simulink model "IdmEstimation_Cogen"  (R2017b)
settings: Solver=FixedStepDiscrete  StartTime=0.0  StopTime=SimTime  FixedStep=0.01  RelTol=1e-3
values from neighbouring files (symbols this model uses):
  BaseMap_CoastAccdiff_Index = (0:0.5:3.5)'    [IdmDev_MdlClassification.m]    (also in IdmParam.mat = [0 0.5 1 1.5 2 2.5 3 3.5])
  BaseMap_CoastSpeed_Index = (5:5:40)'    [IdmDev_MdlClassification.m]    (also in IdmParam.mat = [5 10 15 20 25 30 35 40])
  LrnConfig =     [ModelConfig.mat]
  ModelConfig =     [ModelConfig.mat]
  OnlineConfig =     [ModelConfig.mat]
undefined symbols (not defined in the file or in its folder): acc_veh, dis_veh, ParamCase, vel_veh
libraries: simulink x7
(part 1 of 2)
settings Model: Creator=Kyunghan  LastModifiedBy=Kyunghan
settings DataIOCC: SaveFormat=StructureWithTime
settings OptimizationCC: BlockReduction=off  DefaultParameterBehavior=Inlined  LifeSpan=1
settings DebuggingCC: MultiTaskDSMMsg=warning  FcnCallInpInsideContextMsg=warning  SFExecutionAtInitializationDiag=none
settings HardwareCC: ProdBitPerSizeT=32  ProdBitPerPtrDiffT=32  ProdWordSize=32  ProdHWDeviceType=Specified
settings ModelReferenceCC: PropagateSignalLabelsOutOfModel=off
settings SFSimCC: MATLABDynamicMemAlloc=off
settings RTWCC: SystemTargetFile=ert.tlc  TemplateMakefile=ert_default_tmf  GenerateReport=on  IncludeHyperlinkInReport=on  LaunchReport=on  PortableWordSizes=on  GenerateTraceInfo=on  GenerateTraceReport=on  GenerateTraceReportSl=on  GenerateTraceReportSf=on  GenerateTraceReportEml=on
settings CodeAppCC: ForceParamTrailComments=on  IgnoreCustomStorageClasses=off  OperatorAnnotations=on  SimulinkDataObjDesc=on  SFDataObjDesc=on  InsertBlockDesc=on  StateflowObjectComments=on
settings ERTTargetCC: MultiwordLength=2048  GenerateSampleERTMain=on  MultiInstanceERTCode=on  CodeInterfacePackaging=Reusable function  SupportContinuousTime=on  SupportVariableSizeSignals=on  InlinedParameterPlacement=NonHierarchical  MultiInstanceErrorCode=Warning  RootIOFormat=Structure reference  ERTCustomFileTemplate=example_file_process.tlc  EnableDataOwnership=on  GlobalDataDefinition=InSeparateSourceFile  DataDefinitionFile=Idm_Param.c  GlobalDataReference=InSeparateHeaderFile  DataReferenceFile=Idm_Param.h  ConvertIfToSwitch=off  SuppressUnreachableDefaultCases=off

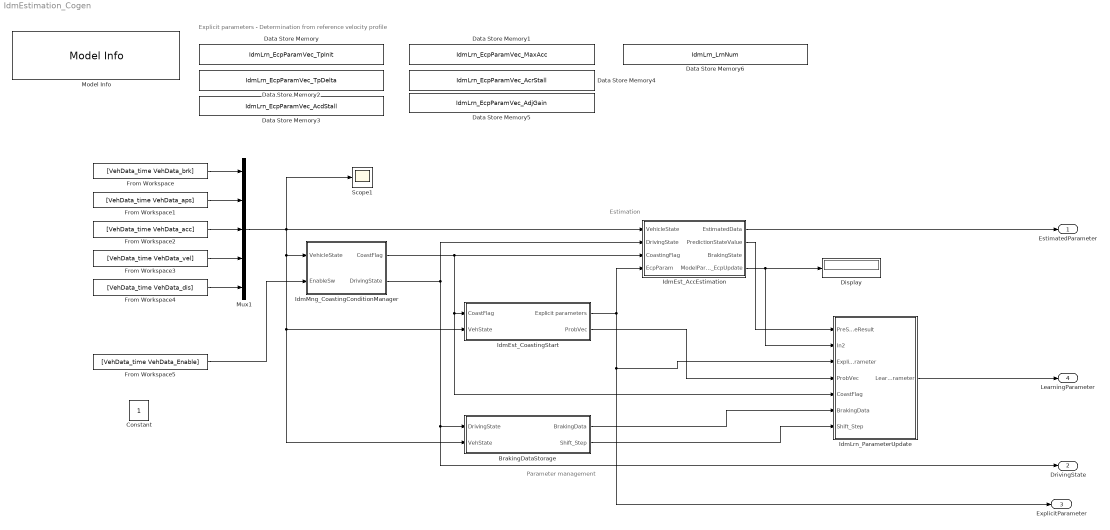
== system IdmEstimation_Cogen ==
  note: Parameter management
  note: Estimation
  note: Explicit parameters - Determination from reference velocity profile
  BrakingDataStorage : Subsystem
      settings: RTWFcnNameOpts=Use subsystem name  RTWFileNameOpts=Use subsystem name
  Constant : Constant  OutDataTypeStr=single
  Data Store Memory : DataStoreMemory  DataStoreName=IdmLrn_EcpParamVec_TpInit  ReadBeforeWriteMsg=warning  WriteAfterWriteMsg=warning  WriteAfterReadMsg=warning  InitialValue=BaseMap_TpShift_Data  ShowAdditionalParam=off  Dimensions=LrnConfig.DataIndexLength  StateMustResolveToSignalObject=on
  Data Store Memory1 : DataStoreMemory  DataStoreName=IdmLrn_EcpParamVec_MaxAcc  ReadBeforeWriteMsg=warning  WriteAfterWriteMsg=warning  WriteAfterReadMsg=warning  InitialValue=BaseMap_MaxAcc_Data  ShowAdditionalParam=off  Dimensions=LrnConfig.DataIndexLength  StateMustResolveToSignalObject=on
  Data Store Memory2 : DataStoreMemory  DataStoreName=IdmLrn_EcpParamVec_TpDelta  ReadBeforeWriteMsg=warning  WriteAfterWriteMsg=warning  WriteAfterReadMsg=warning  InitialValue=BaseMap_TpDelta_Data  ShowAdditionalParam=off  Dimensions=LrnConfig.DataIndexLength  StateMustResolveToSignalObject=on
  Data Store Memory3 : DataStoreMemory  DataStoreName=IdmLrn_EcpParamVec_AcdStall  ReadBeforeWriteMsg=warning  WriteAfterWriteMsg=warning  WriteAfterReadMsg=warning  InitialValue=BaseMap_AccDiff_Data  ShowAdditionalParam=off  Dimensions=LrnConfig.DataIndexLength  StateMustResolveToSignalObject=on
  Data Store Memory4 : DataStoreMemory  DataStoreName=IdmLrn_EcpParamVec_AcrStall  ReadBeforeWriteMsg=warning  WriteAfterWriteMsg=warning  WriteAfterReadMsg=warning  InitialValue=BaseMap_AprStall_Data  ShowAdditionalParam=off  Dimensions=LrnConfig.DataIndexLength  StateMustResolveToSignalObject=on
  Data Store Memory5 : DataStoreMemory  DataStoreName=IdmLrn_EcpParamVec_AdjGain  ReadBeforeWriteMsg=warning  WriteAfterWriteMsg=warning  WriteAfterReadMsg=warning  InitialValue=BaseMap_AdjGain_Data  ShowAdditionalParam=off  Dimensions=LrnConfig.DataIndexLength  StateMustResolveToSignalObject=on
  Data Store Memory6 : DataStoreMemory  DataStoreName=IdmLrn_LrnNum  ReadBeforeWriteMsg=warning  WriteAfterWriteMsg=warning  WriteAfterReadMsg=warning  InitialValue=LrnFacNum  ShowAdditionalParam=off  Dimensions=1  StateMustResolveToSignalObject=on
  Display : Display
  From Workspace : FromWorkspace  VariableName=[VehData_time VehData_brk]  SampleTime=0.01
  From Workspace1 : FromWorkspace  VariableName=[VehData_time VehData_aps]  SampleTime=0.01
  From Workspace2 : FromWorkspace  VariableName=[VehData_time VehData_acc]  SampleTime=0.01
  From Workspace3 : FromWorkspace  VariableName=[VehData_time VehData_vel]  SampleTime=0.01
  From Workspace4 : FromWorkspace  VariableName=[VehData_time VehData_dis]  SampleTime=0.01
  From Workspace5 : FromWorkspace  VariableName=[VehData_time VehData_Enable]  SampleTime=0.01
  IdmEst_AccEstimation : Subsystem
      settings: RTWFcnNameOpts=Use subsystem name  RTWFileNameOpts=Use subsystem name
  IdmEst_CoastingStart : Subsystem
      settings: RTWFcnNameOpts=Use subsystem name  RTWFileNameOpts=Use subsystem name
  IdmLrn_ParameterUpdate : Subsystem
      settings: RTWFcnNameOpts=Use subsystem name  RTWFileNameOpts=Use subsystem name
  IdmMng_CoastingConditionManager : Subsystem
      settings: RTWFcnNameOpts=Use subsystem name  RTWFileNameOpts=Use subsystem name
  Model Info : simulink/Model-Wide Utilities/Model Info  Frame=on  DisplayStringWithTags=|  HorizontalTextAlignment=Left  LeftAlignmentValue=0.02
      | * Model description: %<Description>
      |   1. Description: Estimation model of Idm ver 2
      |   2. Created %<Created> by Kyunghan
      |   3. Modfied %<ModifiedDate> by Kyunghan 
      |   4. Model version:  Ver. 2
  Mux1 : Mux  Inputs=5
  Scope1 : Scope
  EstimatedParameter : Outport
  DrivingState : Outport  Port=2
  ExplicitParameter : Outport  Port=3
  LearningParameter : Outport  Port=4
  wires:
  IdmEst_CoastingStart/1(Explicit parameters) -> IdmEst_AccEstimation/4(EcpParam), ExplicitParameter/1, IdmLrn_ParameterUpdate/3(Explicit parameter)
  Mux1/1 -> Scope1/1, IdmEst_AccEstimation/1(VehicleState), IdmEst_CoastingStart/2(VehState), BrakingDataStorage/2(VehState), IdmMng_CoastingConditionManager/1(VehicleState)
  IdmMng_CoastingConditionManager/1(CoastFlag) -> IdmEst_AccEstimation/3(CoastingFlag), IdmEst_CoastingStart/1(CoastFlag), IdmLrn_ParameterUpdate/5(CoastFlag)
  IdmMng_CoastingConditionManager/2(DrivingState) -> IdmEst_AccEstimation/2(DrivingState), DrivingState/1, BrakingDataStorage/1(DrivingState)
  IdmEst_AccEstimation/1(EstimatedData) -> EstimatedParameter/1
  IdmEst_CoastingStart/2(ProbVec) -> IdmLrn_ParameterUpdate/4(ProbVec)
  BrakingDataStorage/1(BrakingData) -> IdmLrn_ParameterUpdate/6(BrakingData)
  IdmLrn_ParameterUpdate/1(LearningParameter) -> LearningParameter/1
  From Workspace1/1 -> Mux1/2
  From Workspace2/1 -> Mux1/3
  From Workspace/1 -> Mux1/1
  From Workspace3/1 -> Mux1/4
  From Workspace4/1 -> Mux1/5
  IdmEst_AccEstimation/2(PredictionStateValue) -> IdmLrn_ParameterUpdate/1(PreStateResult)
  From Workspace5/1 -> IdmMng_CoastingConditionManager/2(EnableSw)
  IdmEst_AccEstimation/4(ModelParam_EcpUpdate) -> Display/1, IdmLrn_ParameterUpdate/2(In2)
  BrakingDataStorage/2(Shift_Step) -> IdmLrn_ParameterUpdate/7(Shift_Step)

== system IdmEstimation_Cogen/BrakingDataStorage ==
  DrivingState : Inport
  VehState : Inport  Port=2
  Compare To Constant1 : simulink/Logic and Bit Operations/Compare To Constant  relop===  const=OnlineConfig.DriveState.Braking  OutDataTypeStr=boolean
  Start state : Subsystem
  BrakingData : Outport
  Shift_Step : Outport  Port=2
  wires:
  Start state/1(BrakingData) -> BrakingData/1
  DrivingState/1 -> Compare To Constant1/1
  VehState/1 -> Start state/1(veh_state)
  Compare To Constant1/1 -> Start state/Enable
  Start state/2(Out1) -> Shift_Step/1

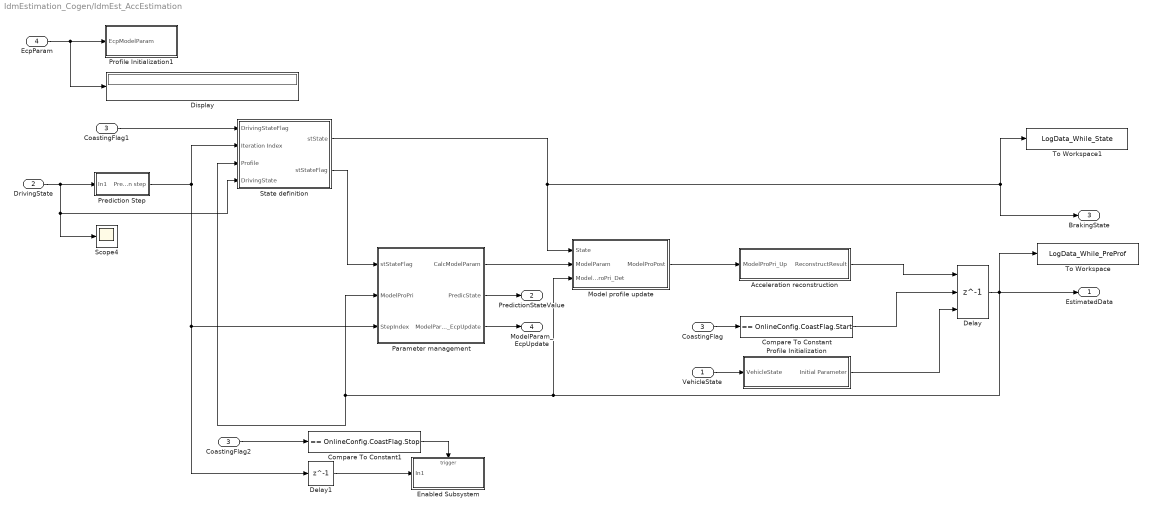
== system IdmEstimation_Cogen/IdmEst_AccEstimation ==
  VehicleState : Inport
  DrivingState : Inport  Port=2
  CoastingFlag : Inport  Port=3
  EcpParam : Inport  Port=4
  Acceleration reconstruction : Subsystem
  CoastingFlag1 : InportShadow  Port=3
  CoastingFlag2 : InportShadow  Port=3
  Compare To Constant : simulink/Logic and Bit Operations/Compare To Constant  relop===  const=OnlineConfig.CoastFlag.Start  OutDataTypeStr=boolean
  Compare To Constant1 : simulink/Logic and Bit Operations/Compare To Constant  relop===  const=OnlineConfig.CoastFlag.Stop  OutDataTypeStr=boolean
  Delay : Delay  DelayLength=1  InitialConditionSource=Input port  InitialCondition=[acc_veh(1) 0 vel_veh(1) vel_veh(1)-ParamCase.VpDiff_Coast dis_veh(1) 0 0]  ExternalReset=Rising
      settings: InputPortMap=u0,r5,p4
  Delay1 : Delay  DelayLength=1
  Display : Display
  Enabled Subsystem : Subsystem  TreatAsAtomicUnit=on
  Model profile update : Subsystem
  Parameter management : Subsystem
  Prediction Step : Subsystem
  Profile Initialization : Subsystem
  Profile Initialization1 : Subsystem
  Scope4 : Scope
  State definition : Subsystem
  To Workspace : ToWorkspace  VariableName=LogData_While_PreProf  SaveFormat=Structure With Time  SampleTime=-1
  To Workspace1 : ToWorkspace  VariableName=LogData_While_State  SaveFormat=Structure With Time  SampleTime=-1
  EstimatedData : Outport  InitialOutput=zeros(1,7)
  PredictionStateValue : Outport  Port=2  InitialOutput=zeros(1,6)
  BrakingState : Outport  Port=3
  ModelParam_EcpUpdate : Outport  Port=4
  wires:
  Compare To Constant/1 -> Delay/2
  Prediction Step/1(Prediction step) -> State definition/2(Iteration Index), Delay1/1, Parameter management/3(StepIndex)
  State definition/2(stStateFlag) -> Parameter management/1(stStateFlag)
  Delay/1 -> To Workspace/1, EstimatedData/1, Model profile update/3(ModelProPri_Det), Parameter management/2(ModelProPri), State definition/3(Profile)
  EcpParam/1 -> Display/1, Profile Initialization1/1(EcpModelParam)
  VehicleState/1 -> Profile Initialization/1(VehicleState)
  Parameter management/1(CalcModelParam) -> Model profile update/2(ModelParam)
  Acceleration reconstruction/1(ReconstructResult) -> Delay/1
  Model profile update/1(ModelProPost) -> Acceleration reconstruction/1(ModelProPri_Up)
  Profile Initialization/1(Initial Parameter) -> Delay/3
  State definition/1(stState) -> BrakingState/1, To Workspace1/1, Model profile update/1(State)
  DrivingState/1 -> State definition/4(DrivingState), Scope4/1, Prediction Step/1(In1)
  Parameter management/2(PredicState) -> PredictionStateValue/1
  CoastingFlag/1 -> Compare To Constant/1
  CoastingFlag1/1 -> State definition/1(DrivingStateFlag)
  Parameter management/3(ModelParam_EcpUpdate) -> ModelParam_EcpUpdate/1
  CoastingFlag2/1 -> Compare To Constant1/1
  Compare To Constant1/1 -> Enabled Subsystem/Trigger
  Delay1/1 -> Enabled Subsystem/1(In1)

== system IdmEstimation_Cogen/IdmEst_CoastingStart ==
  CoastFlag : Inport
  VehState : Inport  Port=2
  Compare To Constant : simulink/Logic and Bit Operations/Compare To Constant  relop===  const=OnlineConfig.CoastFlag.Start  OutDataTypeStr=boolean
  Explicit parameter selection : Subsystem
  Explicit parameters : Outport
  ProbVec : Outport  Port=2
  wires:
  Explicit parameter selection/1(ExplicitParameter) -> Explicit parameters/1
  CoastFlag/1 -> Compare To Constant/1
  VehState/1 -> Explicit parameter selection/1(VehicleState)
  Compare To Constant/1 -> Explicit parameter selection/Trigger
  Explicit parameter selection/2(ProbVec_vel) -> ProbVec/1

== system IdmEstimation_Cogen/IdmLrn_ParameterUpdate ==
  PreStateResult : Inport
  In2 : Inport  Port=2
  Explicit parameter : Inport  Port=3
  ProbVec : Inport  Port=4
  CoastFlag : Inport  Port=5
  BrakingData : Inport  Port=6
  Shift_Step : Inport  Port=7
  Compare To Constant : simulink/Logic and Bit Operations/Compare To Constant  relop===  const=OnlineConfig.CoastFlag.Stop  OutDataTypeStr=boolean
  Compare To Constant1 : simulink/Logic and Bit Operations/Compare To Constant  relop===  const=OnlineConfig.CoastFlag.Stop  OutDataTypeStr=boolean
  End state : Subsystem
  Parameter update : Subsystem
  LearningParameter : Outport
  wires:
  Compare To Constant/1 -> Parameter update/Trigger
  Explicit parameter/1 -> Parameter update/1(ExplicitParameter)
  ProbVec/1 -> Parameter update/3(ProbVec)
  End state/1(LearningParameter) -> Parameter update/2(LearningParameter), LearningParameter/1
  CoastFlag/1 -> Compare To Constant1/1, Compare To Constant/1
  Compare To Constant1/1 -> End state/Trigger
  BrakingData/1 -> End state/1(BrakingDataArry)
  PreStateResult/1 -> Parameter update/4(PreStateResult), End state/3(PreStateResult)
  In2/1 -> Parameter update/5(In5)
  Shift_Step/1 -> End state/2(Shift_Step)

== system IdmEstimation_Cogen/IdmMng_CoastingConditionManager ==
  VehicleState : Inport
  EnableSw : Inport  Port=2
  Chart : Stateflow chart  TreatAsAtomicUnit=on
  Constant : Constant  Value=0
  Selector : Selector  InputPortWidth=OnlineConfig.VehStateSize  IndexOptions=Index vector (dialog)  Indices=OnlineConfig.VehStateIndex.Aps  OutputSizes=1
  Selector1 : Selector  InputPortWidth=OnlineConfig.VehStateSize  IndexOptions=Index vector (dialog)  Indices=OnlineConfig.VehStateIndex.Vel  OutputSizes=1
  Selector2 : Selector  InputPortWidth=OnlineConfig.VehStateSize  IndexOptions=Index vector (dialog)  Indices=OnlineConfig.VehStateIndex.Dis  OutputSizes=1
  Switch : Switch  Threshold=0.5
  Switch1 : Switch  Threshold=0.5
  CoastFlag : Outport
  DrivingState : Outport  Port=2
  wires:
  VehicleState/1 -> Selector2/1, Selector1/1, Selector/1
  Selector/1 -> Chart/1(Aps)
  Selector1/1 -> Chart/2(Vel)
  Chart/2(stCoastFlag) -> Switch1/1
  Chart/1(stDrvState) -> Switch/1
  Selector2/1 -> Chart/3(Dis)
  EnableSw/1 -> Switch1/2, Switch/2
  Switch/1 -> DrivingState/1
  Constant/1 -> Switch/3, Switch1/3
  Switch1/1 -> CoastFlag/1

== system IdmEstimation_Cogen/BrakingDataStorage/Start state ==
  veh_state : Inport
  Enable : EnablePort  StatesWhenEnabling=reset
  MATLAB Function : MATLAB Function  TreatAsAtomicUnit=on
  MATLAB Function1 : MATLAB Function  TreatAsAtomicUnit=on
  Scope : Scope
  Scope1 : Scope
  Selector : Selector  InputPortWidth=5  IndexOptions=Index vector (dialog)  Indices=1  OutputSizes=1
  BrakingData : Outport  InitialOutput=zeros(2000,3)
  Out1 : Outport  Port=2
  wires:
  MATLAB Function/1(BrakingDataOut) -> BrakingData/1
  veh_state/1 -> Selector/1, MATLAB Function/1(veh_state)
  Selector/1 -> Scope/1, MATLAB Function1/1(Brk_Data)
  MATLAB Function1/1(Shift_TimeOut) -> Scope1/1, Out1/1

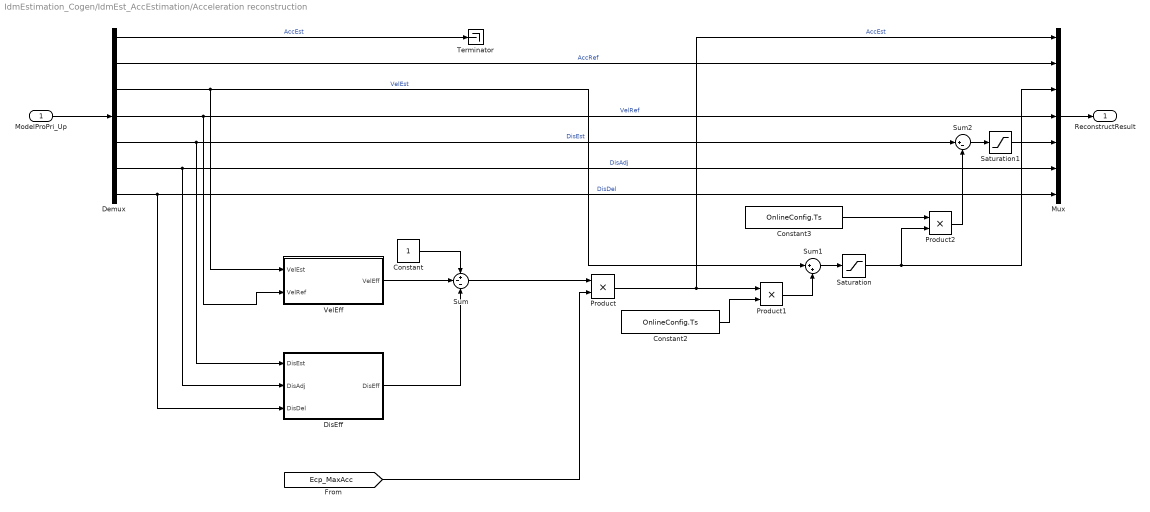
== system IdmEstimation_Cogen/IdmEst_AccEstimation/Acceleration reconstruction ==
  ModelProPri_Up : Inport
  Constant : Constant
  Constant2 : Constant  Value=OnlineConfig.Ts
  Constant3 : Constant  Value=OnlineConfig.Ts
  Demux : Demux  Outputs=7
  DisEff : Subsystem
  Mux : Mux  Inputs=7
  Product : Product
  Product1 : Product
  Product2 : Product
  Saturation : Saturate  UpperLimit=inf  LowerLimit=0.01
  Saturation1 : Saturate  UpperLimit=inf  LowerLimit=0.5001
  Sum : Sum  Inputs=+--
  Sum1 : Sum  Inputs=|++
  Sum2 : Sum  Inputs=|+-
  Terminator : Terminator
  VelEff : Subsystem
  ReconstructResult : Outport
  wires:
  ModelProPri_Up/1 -> Demux/1
  Demux/2 -> Mux/2  "AccRef"
  Mux/1 -> ReconstructResult/1
  Demux/5 -> DisEff/1(DisEst), Sum2/1  "DisEst"
  Demux/6 -> DisEff/2(DisAdj), Mux/6  "DisAdj"
  Demux/7 -> DisEff/3(DisDel), Mux/7  "DisDel"
  Demux/3 -> VelEff/1(VelEst), Sum1/1  "VelEst"
  Demux/4 -> VelEff/2(VelRef), Mux/4  "VelRef"
  VelEff/1(VelEff) -> Sum/2
  DisEff/1(DisEff) -> Sum/3
  Constant/1 -> Sum/1
  Sum/1 -> Product/1
  [Ecp_MaxAcc] -> Product/2
  Product/1 -> Mux/1, Product1/1  "AccEst"
  Constant2/1 -> Product1/2
  Product1/1 -> Sum1/2
  Sum1/1 -> Saturation/1
  Demux/1 -> Terminator/1  "AccEst"
  Constant3/1 -> Product2/1
  Product2/1 -> Sum2/2
  Sum2/1 -> Saturation1/1
  Saturation/1 -> Product2/2, Mux/3
  Saturation1/1 -> Mux/5

== system IdmEstimation_Cogen/IdmEst_AccEstimation/Enabled Subsystem ==
  In1 : Inport
  Trigger : TriggerPort  VariantControl=Variant  PortDimensions=1
  To Workspace : ToWorkspace  VariableName=LogData_Stop_PreSize  SaveFormat=Structure With Time  SampleTime=-1
  wires:
  In1/1 -> To Workspace/1

== system IdmEstimation_Cogen/IdmEst_AccEstimation/Model profile update ==
  State : Inport
  ModelParam : Inport  Port=2
  ModelProPri_Det : Inport  Port=3
  If : If  IfExpression=u1 == 1  ElseIfExpressions=u1 == 2, u1 == 3, u1 == 4, u1 == 5
  Merge : Merge  Inputs=6
  Model profile update - Coast state : Subsystem
  Model profile update - Disadj state : Subsystem
  Model profile update - Initial state : Subsystem
  Model profile update - Term state : Subsystem
  Model profile update - Term state1 : Subsystem
  Model profile update - Veladj state : Subsystem
  ModelProPost : Outport
  wires:
  ModelProPri_Det/1 -> Model profile update - Coast state/1(ModProfPri), Model profile update - Term state1/1(ModProfPri), Model profile update - Term state/1(ModProfPri), Model profile update - Disadj state/1(ModProfPri), Model profile update - Veladj state/1(ModProfPri), Model profile update - Initial state/1(ModProfPri)
  ModelParam/1 -> Model profile update - Initial state/2(ModParam), Model profile update - Veladj state/2(ModParam), Model profile update - Term state/2(ModParam), Model profile update - Disadj state/2(ModParam)
  Merge/1 -> ModelProPost/1
  State/1 -> If/1
  If/4 -> Model profile update - Disadj state/Action
  If/1 -> Model profile update - Coast state/Action
  If/5 -> Model profile update - Term state/Action
  If/2 -> Model profile update - Initial state/Action
  If/3 -> Model profile update - Veladj state/Action
  Model profile update - Coast state/1(ModProf) -> Merge/1
  Model profile update - Initial state/1(ModProf) -> Merge/2
  Model profile update - Veladj state/1(ModProf) -> Merge/3
  Model profile update - Disadj state/1(ModProf) -> Merge/4
  Model profile update - Term state/1(ModProf) -> Merge/5
  If/6 -> Model profile update - Term state1/Action
  Model profile update - Term state1/1(ModProf) -> Merge/6
  [Ecp_AdjGain] -> Model profile update - Disadj state/3(EcpParam_AdjGain)

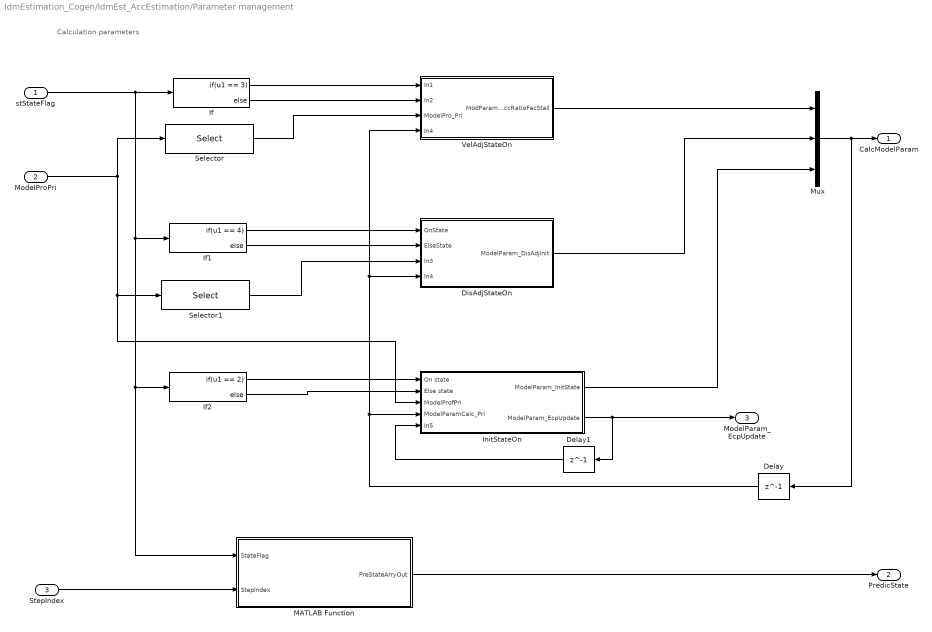
== system IdmEstimation_Cogen/IdmEst_AccEstimation/Parameter management ==
  note: Calculation parameters
  stStateFlag : Inport
  ModelProPri : Inport  Port=2
  StepIndex : Inport  Port=3
  Delay : Delay  DelayLength=1
  Delay1 : Delay  DelayLength=1
  DisAdjStateOn : Subsystem
  If : If  IfExpression=u1 == 3
  If1 : If  IfExpression=u1 == 4
  If2 : If  IfExpression=u1 == 2
  InitStateOn : Subsystem
  MATLAB Function : MATLAB Function  TreatAsAtomicUnit=on
  Mux : Mux  Inputs=3
  Selector : Selector  InputPortWidth=7  IndexOptions=Index vector (dialog)  Indices=[1 3 5]  OutputSizes=1
  Selector1 : Selector  InputPortWidth=7  IndexOptions=Index vector (dialog)  Indices=[1 2]  OutputSizes=1
  VelAdjStateOn : Subsystem
  CalcModelParam : Outport
  PredicState : Outport  Port=2
  ModelParam_EcpUpdate : Outport  Port=3
  wires:
  stStateFlag/1 -> If2/1, MATLAB Function/1(StateFlag), If1/1, If/1
  Mux/1 -> Delay/1, CalcModelParam/1
  Delay/1 -> InitStateOn/4(ModelParamCalc_Pri), VelAdjStateOn/4(In4), DisAdjStateOn/4(In4)
  If2/1 -> InitStateOn/1(On state)
  If2/2 -> InitStateOn/2(Else state)
  ModelProPri/1 -> InitStateOn/3(ModelProfPri), Selector1/1, Selector/1
  InitStateOn/1(ModelParam_InitState) -> Mux/3
  If1/1 -> DisAdjStateOn/1(OnState)
  If1/2 -> DisAdjStateOn/2(ElseState)
  Selector1/1 -> DisAdjStateOn/3(In3)
  DisAdjStateOn/1(ModelParam_DisAdjInit) -> Mux/2
  If/1 -> VelAdjStateOn/1(In1)
  If/2 -> VelAdjStateOn/2(In2)
  Selector/1 -> VelAdjStateOn/3(ModelPro_Pri)
  VelAdjStateOn/1(ModParam_AccRatioFacStall) -> Mux/1
  StepIndex/1 -> MATLAB Function/2(StepIndex)
  MATLAB Function/1(PreStateArryOut) -> PredicState/1
  InitStateOn/2(ModelParam_EcpUpdate) -> ModelParam_EcpUpdate/1, Delay1/1
  Delay1/1 -> InitStateOn/5(In5)

== system IdmEstimation_Cogen/IdmEst_AccEstimation/Prediction Step ==
  In1 : Inport
  Delay : Delay  DelayLength=1
  If : If  IfExpression=u1 == 1
  If Action Subsystem : Subsystem  TreatAsAtomicUnit=on
  If Action Subsystem1 : Subsystem  TreatAsAtomicUnit=on
  Merge : Merge
  Prediction step : Outport
  wires:
  If/1 -> If Action Subsystem/Action
  If/2 -> If Action Subsystem1/Action
  If Action Subsystem/1(Out1) -> Merge/1
  If Action Subsystem1/1(Out1) -> Merge/2
  Merge/1 -> Prediction step/1, Delay/1
  In1/1 -> If/1
  Delay/1 -> If Action Subsystem/1(In1)

== system IdmEstimation_Cogen/IdmEst_AccEstimation/Profile Initialization ==
  VehicleState : Inport
  Constant : Constant  Value=0
  Constant2 : Constant  Value=0
  Constant3 : Constant  Value=0
  Mux : Mux  Inputs=7
  Selector1 : Selector  InputPortWidth=OnlineConfig.VehStateSize  IndexOptions=Index vector (dialog)  Indices=OnlineConfig.VehStateIndex.Vel  OutputSizes=1
  Selector2 : Selector  InputPortWidth=OnlineConfig.VehStateSize  IndexOptions=Index vector (dialog)  Indices=OnlineConfig.VehStateIndex.Dis  OutputSizes=1
  Selector3 : Selector  InputPortWidth=OnlineConfig.VehStateSize  IndexOptions=Index vector (dialog)  Indices=OnlineConfig.VehStateIndex.Acc  OutputSizes=1
  Subsystem : Subsystem
  Initial Parameter : Outport
  wires:
  Constant/1 -> Mux/2
  Subsystem/1(VelRefInit) -> Mux/4
  Constant2/1 -> Mux/6
  Constant3/1 -> Mux/7
  VehicleState/1 -> Selector3/1, Selector2/1, Selector1/1
  Mux/1 -> Initial Parameter/1
  Selector2/1 -> Mux/5
  Selector1/1 -> Subsystem/1(Vel), Mux/3
  Selector3/1 -> Subsystem/2(Acc), Mux/1

== system IdmEstimation_Cogen/IdmEst_AccEstimation/Profile Initialization1 ==
  EcpModelParam : Inport
  Selector : Selector  InputPortWidth=OnlineConfig.EpcParamSize  IndexOptions=Index vector (dialog)  Indices=OnlineConfig.EpcParamIndex.TpInit  OutputSizes=1
  Selector1 : Selector  InputPortWidth=OnlineConfig.EpcParamSize  IndexOptions=Index vector (dialog)  Indices=OnlineConfig.EpcParamIndex.TpStall  OutputSizes=1
  Selector3 : Selector  InputPortWidth=OnlineConfig.EpcParamSize  IndexOptions=Index vector (dialog)  Indices=OnlineConfig.EpcParamIndex.AcrStall  OutputSizes=1
  Selector4 : Selector  InputPortWidth=OnlineConfig.EpcParamSize  IndexOptions=Index vector (dialog)  Indices=OnlineConfig.EpcParamIndex.AccMax  OutputSizes=1
  Selector5 : Selector  InputPortWidth=OnlineConfig.EpcParamSize  IndexOptions=Index vector (dialog)  Indices=OnlineConfig.EpcParamIndex.AdjGain  OutputSizes=1
  tag scope: Ecp_AdjGain=global, Ecp_ArStall=global, Ecp_MaxAcc=global, Ecp_TpDelta=global, Ecp_TpInit=global
  wires:
  EcpModelParam/1 -> Selector1/1, Selector5/1, Selector4/1, Selector3/1, Selector/1
  Selector/1 -> [Ecp_TpInit]
  Selector3/1 -> [Ecp_ArStall]
  Selector1/1 -> [Ecp_TpDelta]
  Selector4/1 -> [Ecp_MaxAcc]
  Selector5/1 -> [Ecp_AdjGain]

== system IdmEstimation_Cogen/IdmEst_AccEstimation/State definition ==
  DrivingStateFlag : Inport
  Iteration Index : Inport  Port=2
  Profile : Inport  Port=3
  DrivingState : Inport  Port=4
  Chart : Stateflow chart  TreatAsAtomicUnit=on
  stState : Outport
  stStateFlag : Outport  Port=2
  wires:
  Profile/1 -> Chart/4(ModelProfile)
  Iteration Index/1 -> Chart/3(IndexTimeStep)
  Chart/1(stState) -> stState/1
  Chart/2(stStateFlag) -> stStateFlag/1
  [Ecp_TpInit] -> Chart/5(Param_Tp_Init)
  [Ecp_TpDelta] -> Chart/6(Param_Tp_Delta)
  [Ecp_ArStall] -> Chart/7(Param_Acr_Stall)
  DrivingStateFlag/1 -> Chart/1(DrvStateFlag)
  DrivingState/1 -> Chart/2(DrivingState)

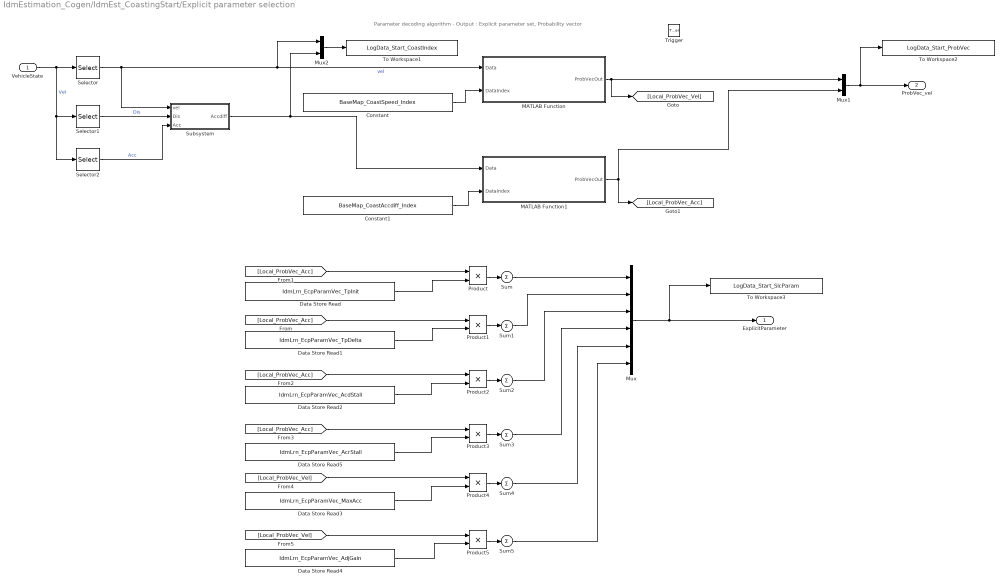
== system IdmEstimation_Cogen/IdmEst_CoastingStart/Explicit parameter selection ==
  note: Parameter decoding algorithm - Output : Explicit parameter set, Probability vector
  VehicleState : Inport
  Trigger : TriggerPort  VariantControl=(inherit)  PortDimensions=1
  Constant : Constant  Value=BaseMap_CoastSpeed_Index
  Constant1 : Constant  Value=BaseMap_CoastAccdiff_Index
  Data Store Read : DataStoreRead  DataStoreName=IdmLrn_EcpParamVec_TpInit
  Data Store Read1 : DataStoreRead  DataStoreName=IdmLrn_EcpParamVec_TpDelta
  Data Store Read2 : DataStoreRead  DataStoreName=IdmLrn_EcpParamVec_AcdStall
  Data Store Read3 : DataStoreRead  DataStoreName=IdmLrn_EcpParamVec_MaxAcc
  Data Store Read4 : DataStoreRead  DataStoreName=IdmLrn_EcpParamVec_AdjGain
  Data Store Read5 : DataStoreRead  DataStoreName=IdmLrn_EcpParamVec_AcrStall
  MATLAB Function : MATLAB Function  TreatAsAtomicUnit=on
  MATLAB Function1 : MATLAB Function  TreatAsAtomicUnit=on
  Mux : Mux  Inputs=6
  Mux1 : Mux  Inputs=2
  Mux2 : Mux  Inputs=2
  Product{,1..5} (6 alike) : Product
  Selector : Selector  InputPortWidth=OnlineConfig.VehStateSize  IndexOptions=Index vector (dialog)  Indices=OnlineConfig.VehStateIndex.Vel  OutputSizes=1
  Selector1 : Selector  InputPortWidth=OnlineConfig.VehStateSize  IndexOptions=Index vector (dialog)  Indices=OnlineConfig.VehStateIndex.Dis  OutputSizes=1
  Selector2 : Selector  InputPortWidth=OnlineConfig.VehStateSize  IndexOptions=Index vector (dialog)  Indices=OnlineConfig.VehStateIndex.Acc  OutputSizes=1
  Subsystem : Subsystem
  Sum{,1..5} (6 alike) : Sum  Inputs=1
  To Workspace1 : ToWorkspace  VariableName=LogData_Start_CoastIndex  SaveFormat=Structure With Time  SampleTime=-1
  To Workspace2 : ToWorkspace  VariableName=LogData_Start_ProbVec  SaveFormat=Structure With Time  SampleTime=-1
  To Workspace3 : ToWorkspace  VariableName=LogData_Start_SlcParam  SaveFormat=Structure With Time  SampleTime=-1
  ExplicitParameter : Outport  InitialOutput=zeros(6,1)
  ProbVec_vel : Outport  Port=2  InitialOutput=-1
  wires:
  Mux/1 -> To Workspace3/1, ExplicitParameter/1
  Constant/1 -> MATLAB Function/2(DataIndex)
  Data Store Read/1 -> Product/2
  MATLAB Function/1(ProbVecOut) -> [Local_ProbVec_Vel], Mux1/1
  VehicleState/1 -> Selector2/1, Selector1/1, Selector/1  "Vel"
  [Local_ProbVec_Acc] -> Product/1
  [Local_ProbVec_Acc] -> Product1/1
  [Local_ProbVec_Acc] -> Product2/1
  [Local_ProbVec_Acc] -> Product3/1
  [Local_ProbVec_Vel] -> Product4/1
  [Local_ProbVec_Vel] -> Product5/1
  Data Store Read1/1 -> Product1/2
  Data Store Read4/1 -> Product5/2
  Data Store Read3/1 -> Product4/2
  Data Store Read5/1 -> Product3/2
  Data Store Read2/1 -> Product2/2
  Product/1 -> Sum/1
  Product1/1 -> Sum1/1
  Product2/1 -> Sum2/1
  Product3/1 -> Sum3/1
  Product4/1 -> Sum4/1
  Product5/1 -> Sum5/1
  Sum/1 -> Mux/1
  Sum1/1 -> Mux/2
  Sum2/1 -> Mux/3
  Sum3/1 -> Mux/4
  Sum4/1 -> Mux/5
  Sum5/1 -> Mux/6
  Selector/1 -> Subsystem/1(vel), Mux2/1, MATLAB Function/1(Data)  "vel"
  Constant1/1 -> MATLAB Function1/2(DataIndex)
  Selector1/1 -> Subsystem/2(Dis)  "Dis"
  Selector2/1 -> Subsystem/3(Acc)  "Acc"
  Subsystem/1(Accdiff) -> Mux2/2, MATLAB Function1/1(Data)
  MATLAB Function1/1(ProbVecOut) -> Mux1/2, [Local_ProbVec_Acc]
  Mux1/1 -> To Workspace2/1, ProbVec_vel/1
  Mux2/1 -> To Workspace1/1

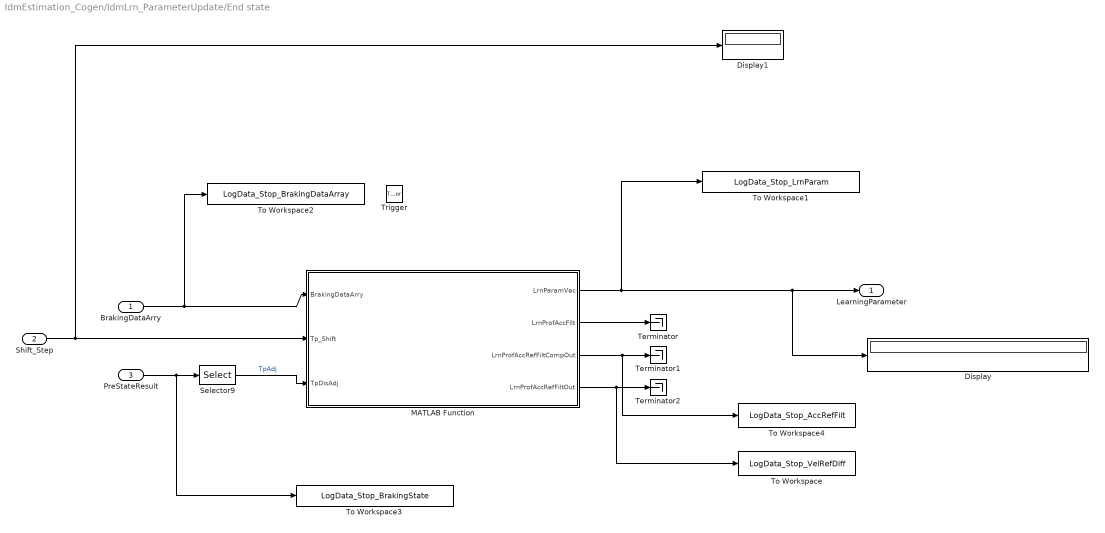
== system IdmEstimation_Cogen/IdmLrn_ParameterUpdate/End state ==
  BrakingDataArry : Inport
  Shift_Step : Inport  Port=2
  PreStateResult : Inport  Port=3
  Trigger : TriggerPort  VariantControl=(inherit)  PortDimensions=1
  Display : Display
  Display1 : Display
  MATLAB Function : MATLAB Function  TreatAsAtomicUnit=on
  Selector9 : Selector  InputPortWidth=ModelConfig.stStateSize  IndexOptions=Index vector (dialog)  Indices=ModelConfig.stState.Disadj  OutputSizes=1
  Terminator : Terminator
  Terminator1 : Terminator
  Terminator2 : Terminator
  To Workspace : ToWorkspace  VariableName=LogData_Stop_VelRefDiff  SaveFormat=Structure With Time  SampleTime=-1
  To Workspace1 : ToWorkspace  VariableName=LogData_Stop_LrnParam  SaveFormat=Structure With Time  SampleTime=-1
  To Workspace2 : ToWorkspace  VariableName=LogData_Stop_BrakingDataArray  SaveFormat=Structure With Time  SampleTime=-1
  To Workspace3 : ToWorkspace  VariableName=LogData_Stop_BrakingState  SaveFormat=Structure With Time  SampleTime=-1
  To Workspace4 : ToWorkspace  VariableName=LogData_Stop_AccRefFilt  SaveFormat=Structure With Time  SampleTime=-1
  LearningParameter : Outport  InitialOutput=zeros(1,6)
  wires:
  BrakingDataArry/1 -> To Workspace2/1, MATLAB Function/1(BrakingDataArry)
  MATLAB Function/1(LrnParamVec) -> To Workspace1/1, Display/1, LearningParameter/1
  PreStateResult/1 -> To Workspace3/1, Selector9/1
  Selector9/1 -> MATLAB Function/3(TpDisAdj)  "TpAdj"
  MATLAB Function/2(LrnProfAccFilt) -> Terminator/1
  MATLAB Function/3(LrnProfAccRefFiltCompOut) -> To Workspace4/1, Terminator1/1
  MATLAB Function/4(LrnProfAccRefFiltOut) -> To Workspace/1, Terminator2/1
  Shift_Step/1 -> Display1/1, MATLAB Function/2(Tp_Shift)

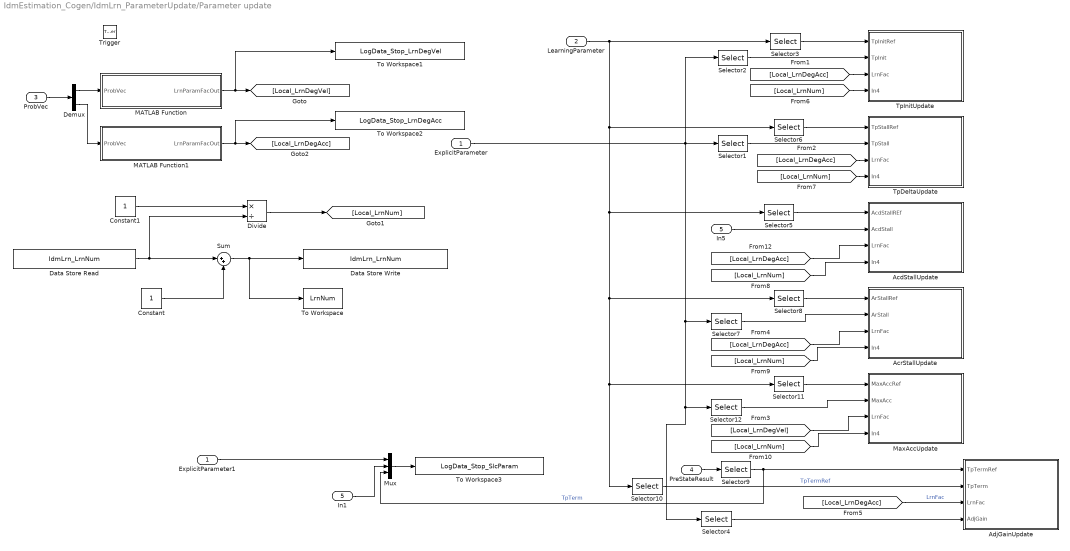
== system IdmEstimation_Cogen/IdmLrn_ParameterUpdate/Parameter update ==
  ExplicitParameter : Inport
  LearningParameter : Inport  Port=2
  ProbVec : Inport  Port=3
  PreStateResult : Inport  Port=4
  In5 : Inport  Port=5
  Trigger : TriggerPort  VariantControl=(inherit)  PortDimensions=1
  AcdStallUpdate : Subsystem
  AcrStallUpdate : Subsystem
  AdjGainUpdate : Subsystem
  Constant : Constant
  Constant1 : Constant
  Data Store Read : DataStoreRead  DataStoreName=IdmLrn_LrnNum
  Data Store Write : DataStoreWrite  DataStoreName=IdmLrn_LrnNum
  Demux : Demux  Outputs=2
  Divide : Product  Inputs=*/
  ExplicitParameter1 : InportShadow
  In1 : InportShadow  Port=5
  MATLAB Function : MATLAB Function  TreatAsAtomicUnit=on
  MATLAB Function1 : MATLAB Function  TreatAsAtomicUnit=on
  MaxAccUpdate : Subsystem
  Mux : Mux  Inputs=3
  Selector1 : Selector  InputPortWidth=OnlineConfig.EpcParamSize  IndexOptions=Index vector (dialog)  Indices=OnlineConfig.EpcParamIndex.TpStall  OutputSizes=1
  Selector10 : Selector  InputPortWidth=OnlineConfig.EpcParamSize  IndexOptions=Index vector (dialog)  Indices=OnlineConfig.EpcParamIndex.AdjGain  OutputSizes=1
  Selector11 : Selector  InputPortWidth=OnlineConfig.EpcParamSize  IndexOptions=Index vector (dialog)  Indices=OnlineConfig.EpcParamIndex.AccMax  OutputSizes=1
  Selector12 : Selector  InputPortWidth=OnlineConfig.EpcParamSize  IndexOptions=Index vector (dialog)  Indices=OnlineConfig.EpcParamIndex.AccMax  OutputSizes=1
  Selector2 : Selector  InputPortWidth=OnlineConfig.EpcParamSize  IndexOptions=Index vector (dialog)  Indices=OnlineConfig.EpcParamIndex.TpInit  OutputSizes=1
  Selector3 : Selector  InputPortWidth=OnlineConfig.EpcParamSize  IndexOptions=Index vector (dialog)  Indices=OnlineConfig.EpcParamIndex.TpInit  OutputSizes=1
  Selector4 : Selector  InputPortWidth=OnlineConfig.EpcParamSize  IndexOptions=Index vector (dialog)  Indices=OnlineConfig.EpcParamIndex.AdjGain  OutputSizes=1
  Selector5 : Selector  InputPortWidth=OnlineConfig.EpcParamSize  IndexOptions=Index vector (dialog)  Indices=OnlineConfig.EpcParamIndex.AcdStall  OutputSizes=1
  Selector6 : Selector  InputPortWidth=OnlineConfig.EpcParamSize  IndexOptions=Index vector (dialog)  Indices=OnlineConfig.EpcParamIndex.TpStall  OutputSizes=1
  Selector7 : Selector  InputPortWidth=OnlineConfig.EpcParamSize  IndexOptions=Index vector (dialog)  Indices=OnlineConfig.EpcParamIndex.AcrStall  OutputSizes=1
  Selector8 : Selector  InputPortWidth=OnlineConfig.EpcParamSize  IndexOptions=Index vector (dialog)  Indices=OnlineConfig.EpcParamIndex.AcrStall  OutputSizes=1
  Selector9 : Selector  InputPortWidth=ModelConfig.stStateSize  IndexOptions=Index vector (dialog)  Indices=ModelConfig.stState.Term  OutputSizes=1
  Sum : Sum  Inputs=|++
  To Workspace : ToWorkspace  VariableName=LrnNum  SaveFormat=Structure With Time  SampleTime=-1
  To Workspace1 : ToWorkspace  VariableName=LogData_Stop_LrnDegVel  SaveFormat=Structure With Time  SampleTime=-1
  To Workspace2 : ToWorkspace  VariableName=LogData_Stop_LrnDegAcc  SaveFormat=Structure With Time  SampleTime=-1
  To Workspace3 : ToWorkspace  VariableName=LogData_Stop_SlcParam  SaveFormat=Structure With Time  SampleTime=-1
  TpDeltaUpdate : Subsystem
  TpInitUpdate : Subsystem
  wires:
  ExplicitParameter/1 -> Selector4/1, Selector12/1, Selector7/1, Selector2/1, Selector1/1
  ProbVec/1 -> Demux/1
  MATLAB Function/1(LrnParamFacOut) -> To Workspace1/1, [Local_LrnDegVel]
  [Local_LrnDegAcc] -> AdjGainUpdate/3(LrnFac)  "LrnFac"
  LearningParameter/1 -> Selector5/1, Selector10/1, Selector11/1, Selector8/1, Selector6/1, Selector3/1
  PreStateResult/1 -> Selector9/1
  Selector10/1 -> AdjGainUpdate/2(TpTerm)  "TpTermRef"
  Selector9/1 -> Mux/3, AdjGainUpdate/1(TpTermRef)  "TpTerm"
  Selector11/1 -> MaxAccUpdate/1(MaxAccRef)
  Selector3/1 -> TpInitUpdate/1(TpInitRef)
  Selector6/1 -> TpDeltaUpdate/1(TpStallRef)
  In5/1 -> AcdStallUpdate/2(AcdStall)
  Selector8/1 -> AcrStallUpdate/1(ArStallRef)
  Selector2/1 -> TpInitUpdate/2(TpInit)
  Selector1/1 -> TpDeltaUpdate/2(TpStall)
  Selector7/1 -> AcrStallUpdate/2(ArStall)
  [Local_LrnDegAcc] -> TpInitUpdate/3(LrnFac)
  [Local_LrnDegAcc] -> TpDeltaUpdate/3(LrnFac)
  [Local_LrnDegAcc] -> AcdStallUpdate/3(LrnFac)
  [Local_LrnDegAcc] -> AcrStallUpdate/3(LrnFac)
  Selector12/1 -> MaxAccUpdate/2(MaxAcc)
  [Local_LrnDegVel] -> MaxAccUpdate/3(LrnFac)
  Data Store Read/1 -> Divide/2, Sum/1
  Constant/1 -> Sum/2
  Sum/1 -> To Workspace/1, Data Store Write/1
  [Local_LrnNum] -> TpInitUpdate/4(In4)
  [Local_LrnNum] -> TpDeltaUpdate/4(In4)
  [Local_LrnNum] -> AcdStallUpdate/4(In4)
  [Local_LrnNum] -> AcrStallUpdate/4(In4)
  [Local_LrnNum] -> MaxAccUpdate/4(In4)
  Selector4/1 -> AdjGainUpdate/4(AdjGain)
  Constant1/1 -> Divide/1
  Divide/1 -> [Local_LrnNum]
  Demux/1 -> MATLAB Function/1(ProbVec)
  Demux/2 -> MATLAB Function1/1(ProbVec)
  MATLAB Function1/1(LrnParamFacOut) -> To Workspace2/1, [Local_LrnDegAcc]
  Selector5/1 -> AcdStallUpdate/1(AcdStallREf)
  ExplicitParameter1/1 -> Mux/1
  In1/1 -> Mux/2
  Mux/1 -> To Workspace3/1

== system IdmEstimation_Cogen/IdmEst_AccEstimation/Acceleration reconstruction/DisEff ==
  DisEst : Inport
  DisAdj : Inport  Port=2
  DisDel : Inport  Port=3
  Constant1 : Constant  Value=ModelConfig.MinDis + ModelConfig.AdjDis
  Divide1 : Product  Inputs=/*
  Math Function1 : Math  Operator=square  SaturateOnIntegerOverflow=on
  Saturation1 : Saturate  UpperLimit=inf  LowerLimit=0.0001
  Sum : Sum  Inputs=3
  DisEff : Outport
  wires:
  Saturation1/1 -> Divide1/1
  Math Function1/1 -> DisEff/1
  Sum/1 -> Divide1/2
  Divide1/1 -> Math Function1/1
  Constant1/1 -> Sum/3
  DisEst/1 -> Saturation1/1
  DisAdj/1 -> Sum/1
  DisDel/1 -> Sum/2

== system IdmEstimation_Cogen/IdmEst_AccEstimation/Acceleration reconstruction/VelEff ==
  VelEst : Inport
  VelRef : Inport  Port=2
  Constant : Constant  Value=ModelConfig.Delta
  Divide : Product  Inputs=*/
  Math Function : Math  Operator=pow  SaturateOnIntegerOverflow=on
  Saturation : Saturate  UpperLimit=inf  LowerLimit=0
  VelEff : Outport
  wires:
  Saturation/1 -> Math Function/1
  Divide/1 -> Saturation/1
  Math Function/1 -> VelEff/1
  Constant/1 -> Math Function/2
  VelRef/1 -> Divide/2
  VelEst/1 -> Divide/1

== system IdmEstimation_Cogen/IdmEst_AccEstimation/Model profile update/Model profile update - Coast state ==
  ModProfPri : Inport
  Action Port : ActionPort  ActionType=then
  Demux : Demux  Outputs=7
  DisAdjCalc : Subsystem
  DisDelCalc : Subsystem
  Mux : Mux  Inputs=7
  RefAccCalc : Subsystem
  RefVelCalc : Subsystem
  Terminator1 : Terminator
  Terminator2 : Terminator
  Terminator3 : Terminator
  ModProf : Outport
  wires:
  ModProfPri/1 -> Demux/1
  Demux/1 -> RefVelCalc/2(AccEst), Mux/1  "AccEst"
  Demux/2 -> Terminator1/1  "AccRef"
  Demux/3 -> RefAccCalc/1(Mod_VelEstPri), Mux/3  "VelEst"
  Demux/4 -> RefVelCalc/1(Mod_VelRefPri)  "VelRef"
  Demux/5 -> RefAccCalc/2(Mod_DisEstPri), Mux/5  "DisEst"
  Demux/6 -> Terminator2/1  "DisAdj"
  RefVelCalc/1(Mod_VelRef) -> Mux/4
  DisAdjCalc/1(Mod_DisAdj) -> Mux/6
  DisDelCalc/1(Mod_DisDel) -> Mux/7
  RefAccCalc/1(Mod_AccRef) -> Mux/2
  Mux/1 -> ModProf/1
  Demux/7 -> Terminator3/1  "DisDel"

== system IdmEstimation_Cogen/IdmEst_AccEstimation/Model profile update/Model profile update - Disadj state ==
  ModProfPri : Inport
  ModParam : Inport  Port=2
  EcpParam_AdjGain : Inport  Port=3
  Action Port : ActionPort  ActionType=elseif
  Demux : Demux  Outputs=7
  DisAdjCalc : Subsystem
  DisDelCalc : Subsystem
  Mux : Mux  Inputs=7
  RefAccCalc : Subsystem
  RefVelCalc : Subsystem
  Terminator : Terminator
  Terminator1 : Terminator
  Terminator2 : Terminator
  ModProf : Outport
  wires:
  ModParam/1 -> RefVelCalc/4(ModParam), DisDelCalc/2(ModelParam)
  Demux/3 -> RefVelCalc/1(Mod_VelEstPri), RefAccCalc/1(Mod_VelEstPri), Mux/3  "VelEst"
  Demux/1 -> Mux/1  "AccEst"
  Demux/6 -> Terminator2/1  "DisAdj"
  Demux/2 -> Terminator1/1  "AccRef"
  ModProfPri/1 -> Demux/1
  Demux/4 -> Terminator/1  "VelRef"
  Demux/5 -> RefAccCalc/2(Mod_DisEstPri), RefVelCalc/2(Mod_DisEstPri), Mux/5, DisAdjCalc/1(Mod_DisEstPri)  "DisEst"
  Mux/1 -> ModProf/1
  DisAdjCalc/1(Mod_DisAdj) -> RefVelCalc/3(Mod_DisAdjPri), Mux/6
  Demux/7 -> DisDelCalc/1(Mod_DisDelPri)  "DisDel"
  DisDelCalc/1(Mod_DisDel) -> Mux/7
  RefAccCalc/1(Mod_AccRef) -> Mux/2
  RefVelCalc/1(Mod_VelRef) -> Mux/4
  EcpParam_AdjGain/1 -> DisDelCalc/3(In3)

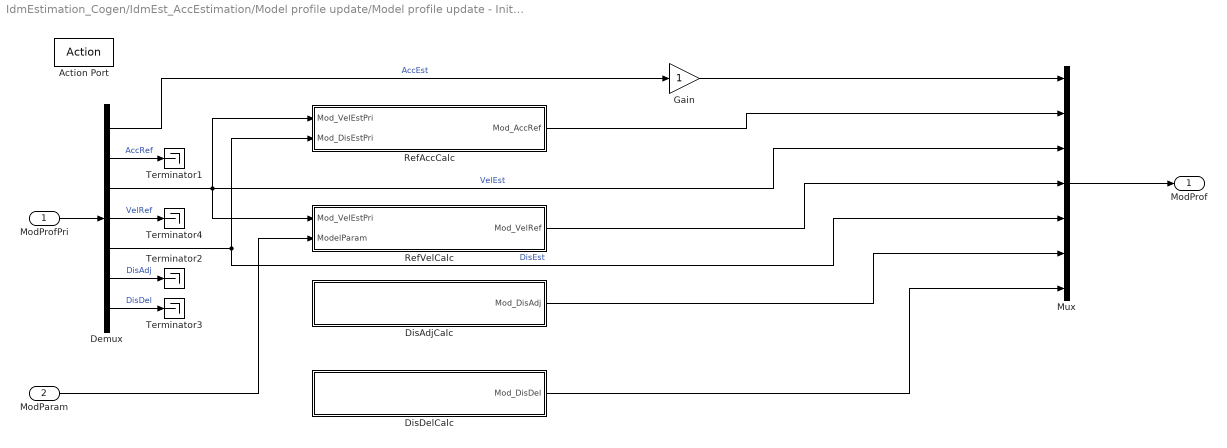
== system IdmEstimation_Cogen/IdmEst_AccEstimation/Model profile update/Model profile update - Initial state ==
  ModProfPri : Inport
  ModParam : Inport  Port=2
  Action Port : ActionPort  ActionType=elseif
  Demux : Demux  Outputs=7
  DisAdjCalc : Subsystem
  DisDelCalc : Subsystem
  Gain : Gain
  Mux : Mux  Inputs=7
  RefAccCalc : Subsystem
  RefVelCalc : Subsystem
  Terminator{1..4} (4 alike) : Terminator
  ModProf : Outport
  wires:
  Mux/1 -> ModProf/1
  RefAccCalc/1(Mod_AccRef) -> Mux/2
  RefVelCalc/1(Mod_VelRef) -> Mux/4
  ModParam/1 -> RefVelCalc/2(ModelParam)
  Demux/7 -> Terminator3/1  "DisDel"
  Demux/6 -> Terminator2/1  "DisAdj"
  Demux/5 -> RefAccCalc/2(Mod_DisEstPri), Mux/5  "DisEst"
  Demux/4 -> Terminator4/1  "VelRef"
  Demux/3 -> RefVelCalc/1(Mod_VelEstPri), RefAccCalc/1(Mod_VelEstPri), Mux/3  "VelEst"
  Demux/2 -> Terminator1/1  "AccRef"
  Demux/1 -> Gain/1  "AccEst"
  ModProfPri/1 -> Demux/1
  DisAdjCalc/1(Mod_DisAdj) -> Mux/6
  DisDelCalc/1(Mod_DisDel) -> Mux/7
  Gain/1 -> Mux/1

== system IdmEstimation_Cogen/IdmEst_AccEstimation/Model profile update/Model profile update - Term state ==
  ModProfPri : Inport
  ModParam : Inport  Port=2
  Action Port : ActionPort  ActionType=elseif
  Demux : Demux  Outputs=7
  DisAdjCalc : Subsystem
  DisDelCalc : Subsystem
  Mux : Mux  Inputs=7
  RefAccCalc : Subsystem
  RefVelCalc : Subsystem
  Terminator : Terminator
  Terminator1 : Terminator
  Terminator2 : Terminator
  ModProf : Outport
  wires:
  Demux/6 -> Terminator2/1  "DisAdj"
  Demux/2 -> Terminator1/1  "AccRef"
  Demux/1 -> DisDelCalc/1(AccEst), Mux/1  "AccEst"
  RefVelCalc/1(Mod_VelRef) -> Mux/4
  DisDelCalc/1(Mod_DisDel) -> Mux/7
  RefAccCalc/1(Mod_AccRef) -> DisDelCalc/2(AccRef), Mux/2
  ModParam/1 -> RefVelCalc/4(ModParam)
  Demux/4 -> Terminator/1  "VelRef"
  Demux/7 -> DisDelCalc/3(Mod_DisDelPri)  "DisDel"
  Mux/1 -> ModProf/1
  Demux/3 -> RefVelCalc/1(Mod_VelEstPri), RefAccCalc/1(Mod_VelEstPri), Mux/3  "VelEst"
  DisAdjCalc/1(Mod_DisAdj) -> RefVelCalc/3(Mod_DisAdjPri), Mux/6
  Demux/5 -> DisAdjCalc/1(Mod_DisEstPri), RefVelCalc/2(Mod_DisEstPri), Mux/5, RefAccCalc/2(Mod_DisEstPri)  "DisEst"
  ModProfPri/1 -> Demux/1

== system IdmEstimation_Cogen/IdmEst_AccEstimation/Model profile update/Model profile update - Term state1 ==
  ModProfPri : Inport
  Action Port : ActionPort  ActionType=else
  ModProf : Outport
  wires:
  ModProfPri/1 -> ModProf/1

== system IdmEstimation_Cogen/IdmEst_AccEstimation/Model profile update/Model profile update - Veladj state ==
  ModProfPri : Inport
  ModParam : Inport  Port=2
  Action Port : ActionPort  ActionType=elseif
  Demux : Demux  Outputs=7
  DisAdjCalc : Subsystem
  DisDelCalc : Subsystem
  Mux : Mux  Inputs=7
  RefAccCalc : Subsystem
  RefVelCalc : Subsystem
  Terminator{,1..3} (4 alike) : Terminator
  ModProf : Outport
  wires:
  DisDelCalc/1(Mod_DisDel) -> Mux/7
  ModParam/1 -> DisAdjCalc/2(ModParam), RefVelCalc/4(ModParam)
  DisAdjCalc/1(Mod_DisAdj) -> Mux/6, RefVelCalc/3(Mod_DisAdjPri)
  Demux/3 -> RefAccCalc/1(Mod_VelEstPri), Mux/3, RefVelCalc/1(Mod_VelEstPri)  "VelEst"
  Demux/1 -> Mux/1  "AccEst"
  Demux/6 -> Terminator1/1  "DisAdj"
  Demux/2 -> Terminator/1  "AccRef"
  ModProfPri/1 -> Demux/1
  Demux/7 -> Terminator2/1  "DisDel"
  Demux/5 -> RefAccCalc/2(Mod_DisEstPri), RefVelCalc/2(Mod_DisEstPri), Mux/5, DisAdjCalc/1(Mod_DisEstPri)  "DisEst"
  RefAccCalc/1(Mod_AccRef) -> Mux/2
  Mux/1 -> ModProf/1
  RefVelCalc/1(Mod_VelRef) -> Mux/4
  Demux/4 -> Terminator3/1  "VelRef"

== system IdmEstimation_Cogen/IdmEst_AccEstimation/Parameter management/DisAdjStateOn ==
  OnState : Inport
  ElseState : Inport  Port=2
  In3 : Inport  Port=3
  In4 : Inport  Port=4
  If Action Subsystem2 : Subsystem  TreatAsAtomicUnit=on
  If Action Subsystem3 : Subsystem  TreatAsAtomicUnit=on
  Merge1 : Merge  InitialOutput=0
  Selector4 : Selector  InputPortWidth=OnlineConfig.CalcParamSize  IndexOptions=Index vector (dialog)  Indices=OnlineConfig.CalcParamIndex.AccdDisAdj  OutputSizes=1
  ModelParam_DisAdjInit : Outport
  wires:
  In3/1 -> If Action Subsystem3/1(ModelProPri)
  If Action Subsystem3/1(ModelParam_DisAdjInit) -> Merge1/1
  Merge1/1 -> ModelParam_DisAdjInit/1  "ModelParam_DisAdjInit"
  ElseState/1 -> If Action Subsystem2/Action
  OnState/1 -> If Action Subsystem3/Action
  If Action Subsystem2/1(Out1) -> Merge1/2
  Selector4/1 -> If Action Subsystem2/1(In1)
  In4/1 -> Selector4/1

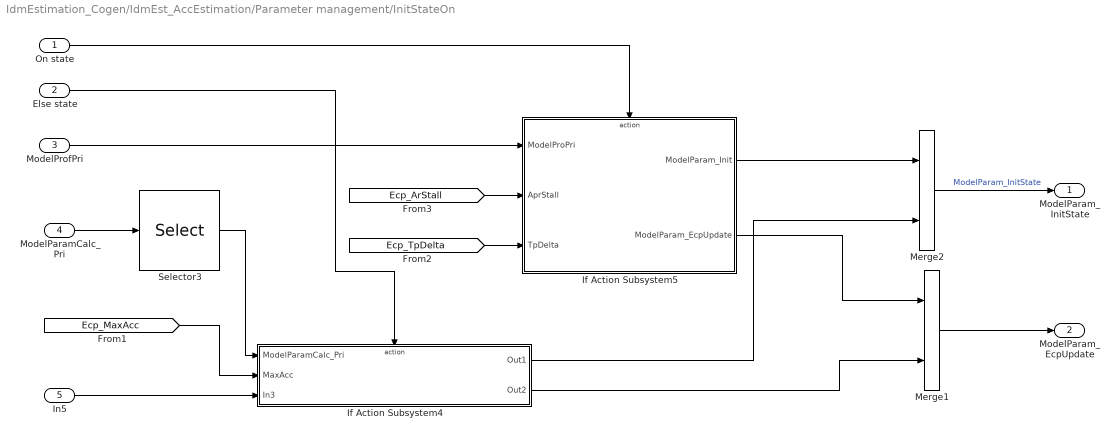
== system IdmEstimation_Cogen/IdmEst_AccEstimation/Parameter management/InitStateOn ==
  On state : Inport
  Else state : Inport  Port=2
  ModelProfPri : Inport  Port=3
  ModelParamCalc_Pri : Inport  Port=4
  In5 : Inport  Port=5
  If Action Subsystem4 : Subsystem  TreatAsAtomicUnit=on
  If Action Subsystem5 : Subsystem  TreatAsAtomicUnit=on
  Merge1 : Merge  InitialOutput=0
  Merge2 : Merge  InitialOutput=0
  Selector3 : Selector  InputPortWidth=OnlineConfig.CalcParamSize  IndexOptions=Index vector (dialog)  Indices=[OnlineConfig.CalcParamIndex.VelRatio OnlineConfig.CalcParamIndex.AccdStall]  OutputSizes=1
  ModelParam_InitState : Outport
  ModelParam_EcpUpdate : Outport  Port=2
  wires:
  ModelParamCalc_Pri/1 -> Selector3/1
  On state/1 -> If Action Subsystem5/Action
  If Action Subsystem4/1(Out1) -> Merge2/2
  Selector3/1 -> If Action Subsystem4/1(ModelParamCalc_Pri)
  Else state/1 -> If Action Subsystem4/Action
  If Action Subsystem5/1(ModelParam_Init) -> Merge2/1
  Merge2/1 -> ModelParam_InitState/1  "ModelParam_InitState"
  [Ecp_ArStall] -> If Action Subsystem5/2(AprStall)
  [Ecp_TpDelta] -> If Action Subsystem5/3(TpDelta)
  [Ecp_MaxAcc] -> If Action Subsystem4/2(MaxAcc)
  ModelProfPri/1 -> If Action Subsystem5/1(ModelProPri)
  If Action Subsystem5/2(ModelParam_EcpUpdate) -> Merge1/1
  Merge1/1 -> ModelParam_EcpUpdate/1
  In5/1 -> If Action Subsystem4/3(In3)
  If Action Subsystem4/2(Out2) -> Merge1/2

== system IdmEstimation_Cogen/IdmEst_AccEstimation/Parameter management/VelAdjStateOn ==
  In1 : Inport
  In2 : Inport  Port=2
  ModelPro_Pri : Inport  Port=3
  In4 : Inport  Port=4
  If Action Subsystem : Subsystem  TreatAsAtomicUnit=on
  If Action Subsystem1 : Subsystem  TreatAsAtomicUnit=on
  Merge : Merge  InitialOutput=[0 0 0]
  Selector5 : Selector  InputPortWidth=OnlineConfig.CalcParamSize  IndexOptions=Index vector (dialog)  Indices=[OnlineConfig.CalcParamIndex.AccrStall OnlineConfig.CalcParamIndex.VelStall OnlineConfig.CalcParamIndex.DisStall]  OutputSizes=1
  ModParam_AccRatioFacStall : Outport
  wires:
  In4/1 -> Selector5/1
  Merge/1 -> ModParam_AccRatioFacStall/1  "ModParam_AccRatioFacStall"
  ModelPro_Pri/1 -> If Action Subsystem/1(ModelProPri)
  If Action Subsystem/1(ModelParam_VelAdjInit) -> Merge/1
  If Action Subsystem1/1(Out1) -> Merge/2
  In1/1 -> If Action Subsystem/Action
  Selector5/1 -> If Action Subsystem1/1(In1)
  In2/1 -> If Action Subsystem1/Action
  [Ecp_MaxAcc] -> If Action Subsystem/2(MaxAcc)

== system IdmEstimation_Cogen/IdmEst_AccEstimation/Prediction Step/If Action Subsystem ==
  In1 : Inport
  Action Port : ActionPort  ActionType=then
  Constant : Constant
  Sum : Sum  Inputs=|++
  Out1 : Outport
  wires:
  Constant/1 -> Sum/1
  Sum/1 -> Out1/1
  In1/1 -> Sum/2

== system IdmEstimation_Cogen/IdmEst_AccEstimation/Prediction Step/If Action Subsystem1 ==
  Action Port : ActionPort  ActionType=else
  Constant : Constant  Value=0
  Out1 : Outport
  wires:
  Constant/1 -> Out1/1

== system IdmEstimation_Cogen/IdmEst_AccEstimation/Profile Initialization/Subsystem ==
  Vel : Inport
  Acc : Inport  Port=2
  Constant1 : Constant
  Constant2 : Constant  Value=1/ModelConfig.Delta
  Divide : Product  Inputs=*/
  Divide1 : Product  Inputs=*/
  Math Function : Math  Operator=pow  SaturateOnIntegerOverflow=on
  Sum : Sum  Inputs=|+-
  VelRefInit : Outport
  wires:
  Vel/1 -> Divide/1
  Acc/1 -> Divide1/1
  Divide/1 -> VelRefInit/1
  [Ecp_MaxAcc] -> Divide1/2
  Constant1/1 -> Sum/1
  Divide1/1 -> Sum/2
  Sum/1 -> Math Function/1
  Constant2/1 -> Math Function/2
  Math Function/1 -> Divide/2

== system IdmEstimation_Cogen/IdmEst_CoastingStart/Explicit parameter selection/Subsystem ==
  note: -0.5*tmpLoc_Mod_vel_est(index_curstep).^2/(tmpLoc_Mod_dis_est(index_curstep) - ModelConfig.StopDis);
  vel : Inport
  Dis : Inport  Port=2
  Acc : Inport  Port=3
  Constant1 : Constant  Value=ModelConfig.StopDis
  Constant2 : Constant  Value=-0.5
  Product1 : Product
  Product2 : Product  Inputs=**/
  Sum : Sum  Inputs=|+-
  Sum1 : Sum  Inputs=|+-
  Accdiff : Outport
  wires:
  Constant1/1 -> Sum/2
  Sum/1 -> Product2/3
  Dis/1 -> Sum/1
  Product2/1 -> Sum1/2
  Constant2/1 -> Product2/1
  vel/1 -> Product1/2, Product1/1
  Product1/1 -> Product2/2
  Acc/1 -> Sum1/1
  Sum1/1 -> Accdiff/1

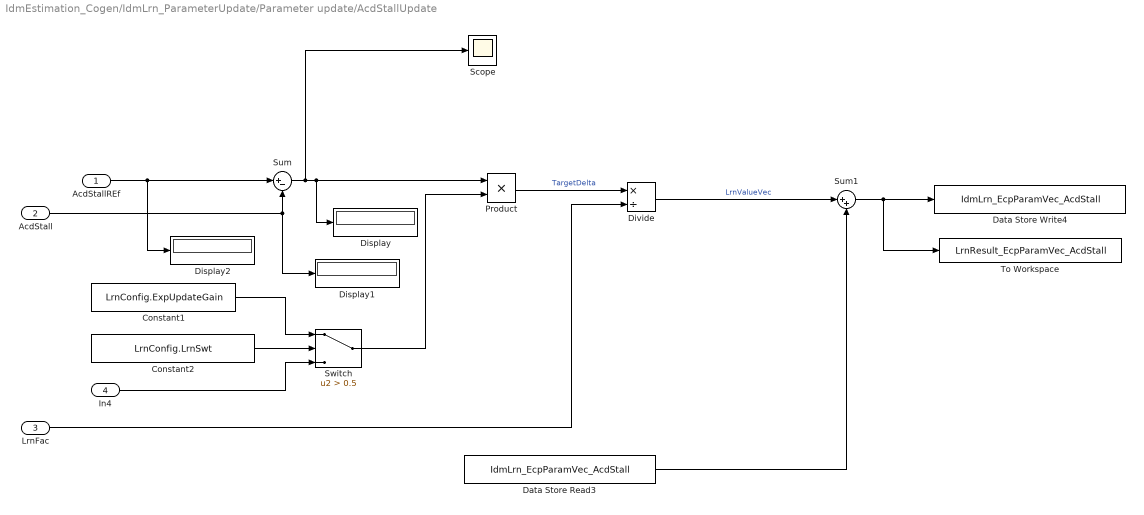
== system IdmEstimation_Cogen/IdmLrn_ParameterUpdate/Parameter update/AcdStallUpdate ==
  AcdStallREf : Inport
  AcdStall : Inport  Port=2
  LrnFac : Inport  Port=3
  In4 : Inport  Port=4
  Constant1 : Constant  Value=LrnConfig.ExpUpdateGain
  Constant2 : Constant  Value=LrnConfig.LrnSwt
  Data Store Read3 : DataStoreRead  DataStoreName=IdmLrn_EcpParamVec_AcdStall
  Data Store Write4 : DataStoreWrite  DataStoreName=IdmLrn_EcpParamVec_AcdStall
  Display : Display
  Display1 : Display
  Display2 : Display
  Divide : Product  Inputs=*/
  Product : Product
  Scope : Scope
  Sum : Sum  Inputs=|+-
  Sum1 : Sum  Inputs=|++
  Switch : Switch  Criteria=u2 > Threshold  Threshold=0.5
  To Workspace : ToWorkspace  VariableName=LrnResult_EcpParamVec_AcdStall  SaveFormat=Structure With Time  SampleTime=-1
  wires:
  Product/1 -> Divide/1  "TargetDelta"
  Sum/1 -> Scope/1, Display/1, Product/1
  AcdStall/1 -> Display1/1, Sum/2
  Switch/1 -> Product/2
  AcdStallREf/1 -> Display2/1, Sum/1
  LrnFac/1 -> Divide/2
  Divide/1 -> Sum1/1  "LrnValueVec"
  Data Store Read3/1 -> Sum1/2
  Sum1/1 -> To Workspace/1, Data Store Write4/1
  Constant2/1 -> Switch/2
  In4/1 -> Switch/3
  Constant1/1 -> Switch/1

== system IdmEstimation_Cogen/IdmLrn_ParameterUpdate/Parameter update/AcrStallUpdate ==
  ArStallRef : Inport
  ArStall : Inport  Port=2
  LrnFac : Inport  Port=3
  In4 : Inport  Port=4
  Constant1 : Constant  Value=LrnConfig.ExpUpdateGain
  Constant2 : Constant  Value=LrnConfig.LrnSwt
  Data Store Read1 : DataStoreRead  DataStoreName=IdmLrn_EcpParamVec_AcrStall
  Data Store Write : DataStoreWrite  DataStoreName=IdmLrn_EcpParamVec_AcrStall
  Display : Display
  Divide : Product  Inputs=*/
  Product : Product
  Sum : Sum  Inputs=|+-
  Sum1 : Sum  Inputs=|++
  Switch : Switch  Criteria=u2 > Threshold  Threshold=0.5
  To Workspace : ToWorkspace  VariableName=LrnResult_EcpParamVec_AcrStall  SaveFormat=Structure With Time  SampleTime=-1
  wires:
  Sum1/1 -> To Workspace/1, Data Store Write/1
  Data Store Read1/1 -> Sum1/2
  Divide/1 -> Sum1/1  "LrnValueVec"
  LrnFac/1 -> Divide/2
  ArStallRef/1 -> Sum/1
  Switch/1 -> Product/2
  ArStall/1 -> Sum/2
  Sum/1 -> Display/1, Product/1
  Product/1 -> Divide/1  "TargetDelta"
  Constant2/1 -> Switch/2
  In4/1 -> Switch/3
  Constant1/1 -> Switch/1

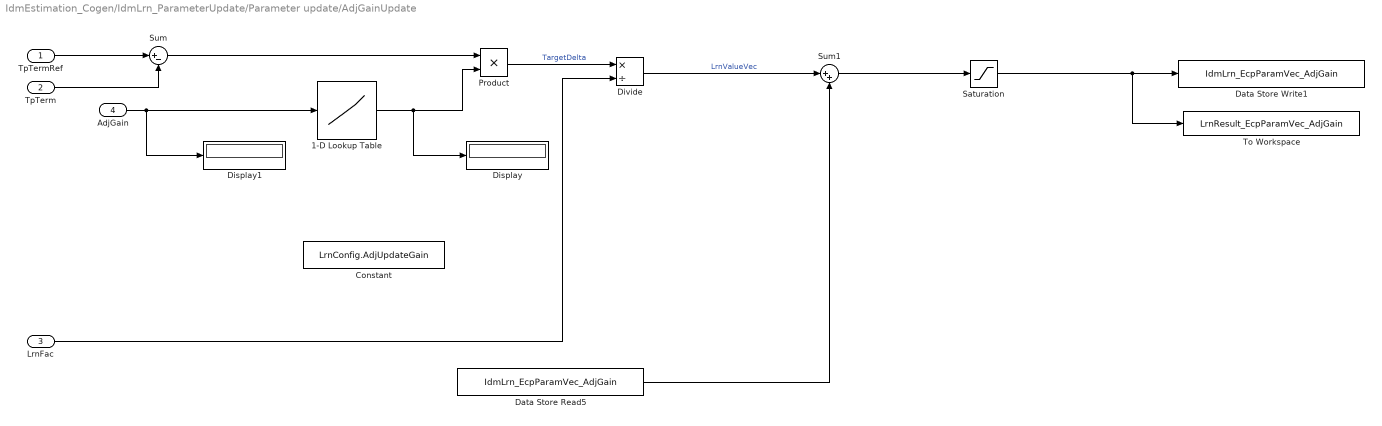
== system IdmEstimation_Cogen/IdmLrn_ParameterUpdate/Parameter update/AdjGainUpdate ==
  TpTermRef : Inport
  TpTerm : Inport  Port=2
  LrnFac : Inport  Port=3
  AdjGain : Inport  Port=4
  1-D Lookup Table : Lookup_n-D  NumberOfTableDimensions=1  BreakpointsForDimension1=[0.005 0.5]  Table=[1e-5 5e-4]  InternalRulePriority=Speed  RndMeth=Simplest  InputSameDT=on
  Constant : Constant  Value=LrnConfig.AdjUpdateGain
  Data Store Read5 : DataStoreRead  DataStoreName=IdmLrn_EcpParamVec_AdjGain
  Data Store Write1 : DataStoreWrite  DataStoreName=IdmLrn_EcpParamVec_AdjGain
  Display : Display
  Display1 : Display
  Divide : Product  Inputs=*/
  Product : Product
  Saturation : Saturate  LowerLimit=0.005
  Sum : Sum  Inputs=|+-
  Sum1 : Sum  Inputs=|++
  To Workspace : ToWorkspace  VariableName=LrnResult_EcpParamVec_AdjGain  SaveFormat=Structure With Time  SampleTime=-1
  wires:
  Product/1 -> Divide/1  "TargetDelta"
  Sum/1 -> Product/1
  TpTerm/1 -> Sum/2
  1-D Lookup Table/1 -> Display/1, Product/2
  TpTermRef/1 -> Sum/1
  LrnFac/1 -> Divide/2
  Divide/1 -> Sum1/1  "LrnValueVec"
  Data Store Read5/1 -> Sum1/2
  Sum1/1 -> Saturation/1
  Saturation/1 -> To Workspace/1, Data Store Write1/1
  AdjGain/1 -> Display1/1, 1-D Lookup Table/1
